simulink subsystem "GeneratorGam_ref_SubSystem"  (R2020b)
settings: Solver=VariableStepAuto  StartTime=0.0  StopTime=10.0  RelTol=1e-3
undefined symbols (not defined in the file or in its folder): r, Ts
settings Model: Creator=umberto  LastModifiedBy=umberto

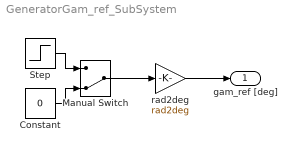
== system GeneratorGam_ref_SubSystem ==
  Constant : Constant  Value=0  SampleTime=Ts
  Manual Switch : ManualSwitch  CurrentSetting=0
  Step : Step  Time=0  After=0.1/r  SampleTime=Ts
  rad2deg : Gain  Gain=rad2deg
  gam_ref [deg] : Outport
  wires:
  rad2deg/1 -> gam_ref [deg]/1
  Step/1 -> Manual Switch/1
  Constant/1 -> Manual Switch/2
  Manual Switch/1 -> rad2deg/1
